simulink model "Lab5_1"  (R2024a)
settings: Solver=VariableStepAuto  StartTime=0.0  StopTime=10  RelTol=1e-3
settings Model: Creator=user  LastModifiedBy=user

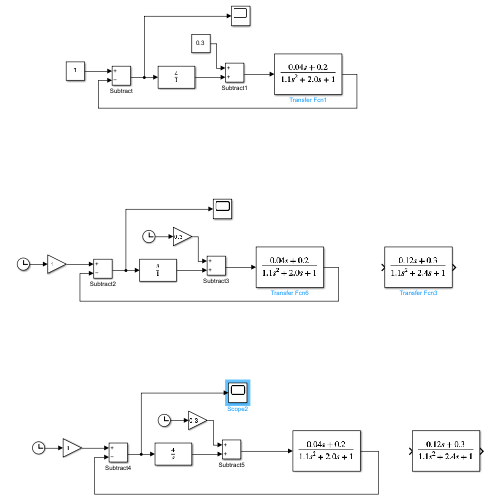
[thumbnail: Simulink's stored preview of the top-level diagram]
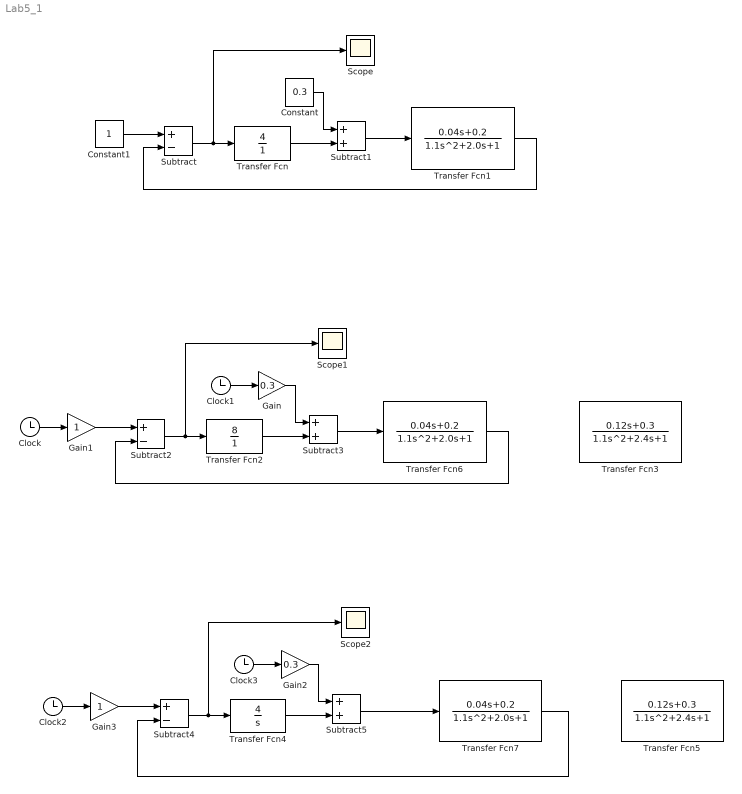
== system Lab5_1 ==
  Clock{,1..3} (4 alike) : Clock
  Constant : Constant  Value=0.3
  Constant1 : Constant
  Gain : Gain  Gain=0.3
  Gain1 : Gain
  Gain2 : Gain  Gain=0.3
  Gain3 : Gain
  Scope : Scope
  Scope1 : Scope
  Scope2 : Scope
  Subtract : Sum  Inputs=+-
  Subtract1 : Sum
  Subtract2 : Sum  Inputs=+-
  Subtract3 : Sum
  Subtract4 : Sum  Inputs=+-
  Subtract5 : Sum
  Transfer Fcn : TransferFcn  Numerator=[4]  Denominator=[1]
  Transfer Fcn1 : TransferFcn  Numerator=[0.04 0.2]  Denominator=[1.1 2.0 1]
  Transfer Fcn2 : TransferFcn  Numerator=[8]  Denominator=[1]
  Transfer Fcn3 : TransferFcn  Numerator=[0.12 0.3]  Denominator=[1.1 2.4 1]
  Transfer Fcn4 : TransferFcn  Numerator=[4]  Denominator=[1 0]
  Transfer Fcn5 : TransferFcn  Numerator=[0.12 0.3]  Denominator=[1.1 2.4 1]
  Transfer Fcn6 : TransferFcn  Numerator=[0.04 0.2]  Denominator=[1.1 2.0 1]
  Transfer Fcn7 : TransferFcn  Numerator=[0.04 0.2]  Denominator=[1.1 2.0 1]
  wires:
  Constant1/1 -> Subtract/1
  Transfer Fcn1/1 -> Subtract/2
  Subtract/1 -> Scope/1, Transfer Fcn/1
  Transfer Fcn/1 -> Subtract1/2
  Constant/1 -> Subtract1/1
  Subtract1/1 -> Transfer Fcn1/1
  Subtract3/1 -> Transfer Fcn6/1
  Gain/1 -> Subtract3/1
  Transfer Fcn2/1 -> Subtract3/2
  Subtract2/1 -> Transfer Fcn2/1, Scope1/1
  Transfer Fcn6/1 -> Subtract2/2
  Gain1/1 -> Subtract2/1
  Clock/1 -> Gain1/1
  Clock1/1 -> Gain/1
  Clock3/1 -> Gain2/1
  Clock2/1 -> Gain3/1
  Gain3/1 -> Subtract4/1
  Transfer Fcn7/1 -> Subtract4/2
  Subtract4/1 -> Scope2/1, Transfer Fcn4/1
  Transfer Fcn4/1 -> Subtract5/2
  Gain2/1 -> Subtract5/1
  Subtract5/1 -> Transfer Fcn7/1
